simulink model "Full_wave_rectifier_RLload"  (R2015b)
settings: Solver=ode45  StartTime=0.0  StopTime=0.5  FixedStep=50e-6  RelTol=1e-3
InitFcn:
  | Vm=339.4;
libraries: powerlib x12
settings Model: Creator=VENKAT  LastModifiedBy=Nikhil
settings DataIOCC: SaveFormat=Array
settings DebuggingCC: SolverPrmCheckMsg=warning
settings HardwareCC: ProdBitPerPointer=32  ProdLargestAtomicFloat=None  ProdIntDivRoundTo=Undefined  ProdEndianess=Unspecified  ProdWordSize=32  ProdHWDeviceType=32-bit Generic
settings GRTTargetCC: GeneratePreprocessorConditionals=Disable all
settings ConfigComp: CovModelRefEnable=Off  CovSFcnEnable=off

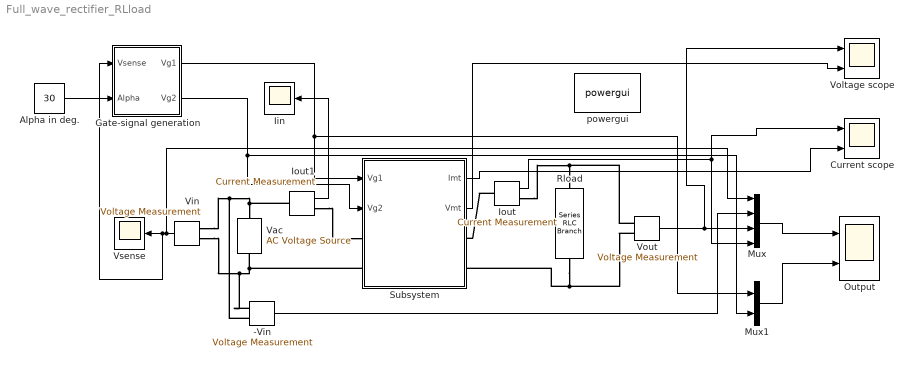
== system Full_wave_rectifier_RLload ==
  -Vin : powerlib/Measurements/Voltage Measurement  PhasorSimulation=off  OutputType=Complex  PSBequivalent=0
  Alpha in deg. : Constant  Value=30
  Current scope : Scope  NumInputPorts=2
  Gate-signal generation : Subsystem
  Iin : Scope
  Iout : powerlib/Measurements/Current Measurement  PhasorSimulation=off  OutputType=Complex  PSBequivalent=0
  Iout1 : powerlib/Measurements/Current Measurement  PhasorSimulation=off  OutputType=Complex  PSBequivalent=0
  Mux : Mux
  Mux1 : Mux  Inputs=2
  Output : Scope  NumInputPorts=2
  Rload : powerlib/Elements/Series RLC Branch  LConnTagsString=__new0  RConnTagsString=__new0  BranchType=RL  Resistance=1  Inductance=1e-2  SetiL0=off  InitialCurrent=0  Capacitance=1e-6  Setx0=off  InitialVoltage=0  Measurements=None
  Subsystem : Subsystem
  Vac : powerlib/Electrical Sources/AC Voltage Source  Amplitude=Vm  Phase=0  Frequency=50  SampleTime=0  Measurements=None  BusType=swing  Pref=10e3  Qref=0  Qmin=-inf  Qmax=+inf
  Vin : powerlib/Measurements/Voltage Measurement  PhasorSimulation=off  OutputType=Complex  PSBequivalent=0
  Voltage scope : Scope  NumInputPorts=2
  Vout : powerlib/Measurements/Voltage Measurement  PhasorSimulation=off  OutputType=Complex  PSBequivalent=0
  Vsense : Scope
  powergui : powerlib/powergui  Priority=1  SimulationMode=Continuous  SolverType=Tustin  SampleTime=50e-6  frequency=60  SPID=on  DisableSnubberDevices=off  DisableRonSwitches=off  DisableVfSwitches=off  SwTol=0  DisplayEquations=off  Interpol=off  ExternalGateDelay=off  methode=off  Ts=0  FunctionMessages=off  echomessages=off  HookPort=off  EnableUseOfTLC=off  x0status=blocks  frequencyindice=50  Pbase=100e6  ErrMax=1e-4  Iterations=50  UnitsV=kV  UnitsW=MW  buscounter=0  RestoreLinks=warning  ResistiveCurrentMeasurement=off  Frange=[0:2:500]  Ylog=off  Xlog=on  ShowGrid=off  save=off  variable=ZData  structure=0  ZoomFFT=off  StartTime=0.0  cycles=1  DisplayStyle=1  fundamental=60  FreqAxis=off  MaxFrequency=1000  frequencyindicesteady=1  RmsSteady=1  display=off
  wires:
  Vin/1 -> Mux/1, Gate-signal generation/1(Vsense), Vsense/1
  Alpha in deg./1 -> Gate-signal generation/2(Alpha)
  Mux/1 -> Output/1
  Gate-signal generation/1(Vg1) -> Mux1/1, Subsystem/1(Vg1)
  Gate-signal generation/2(Vg2) -> Mux1/2, Subsystem/2(Vg2)
  Iout/1 -> Mux/4, Current scope/1
  Vout/1 -> Voltage scope/1, Mux/3
  -Vin/1 -> Mux/2
  Mux1/1 -> Output/2
  Subsystem/1(Imt) -> Current scope/2
  Subsystem/2(Vmt) -> Voltage scope/2
  Iout1/1 -> Iin/1
  connections:
  Vin/LConn1 -- -Vin/LConn2 -- Iout1/LConn1 -- Vac/RConn1
  Rload/RConn1 -- Vout/LConn2 -- Subsystem/RConn2
  Vout/LConn1 -- Iout/RConn1 -- Rload/LConn1
  Vin/LConn2 -- -Vin/LConn1 -- Subsystem/LConn2 -- Vac/LConn1
  Iout/LConn1 -- Subsystem/RConn1
  Iout1/RConn1 -- Subsystem/LConn1

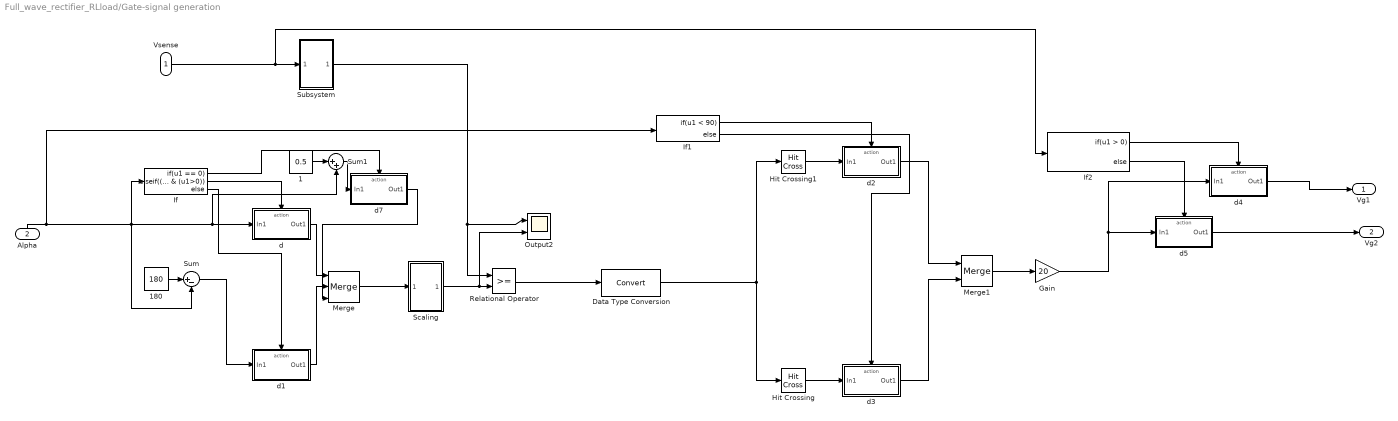
== system Full_wave_rectifier_RLload/Gate-signal generation ==
  Vsense : Inport
  Alpha : Inport  Port=2
  1 : Constant  Value=0.5
  180 : Constant  Value=180
  Data Type Conversion : DataTypeConversion
  Gain : Gain  Gain=20
  Hit Crossing : HitCross  HitCrossingOffset=1e-5  HitCrossingDirection=falling
  Hit Crossing1 : HitCross  HitCrossingDirection=rising
  If : If  IfExpression=u1 == 0  ElseIfExpressions=(u1 < 90) & (u1>0)
  If1 : If  IfExpression=u1 < 90
  If2 : If
  Merge : Merge  Inputs=3
  Merge1 : Merge
  Output2 : Scope  NumInputPorts=2
  Relational Operator : RelationalOperator  OutDataTypeStr=boolean
  Scaling : Subsystem
  Subsystem : Subsystem
  Sum : Sum  Inputs=|+-
  Sum1 : Sum  Inputs=|++
  d : Subsystem  TreatAsAtomicUnit=on
  d1 : Subsystem  TreatAsAtomicUnit=on
  d2 : Subsystem  TreatAsAtomicUnit=on
  d3 : Subsystem  TreatAsAtomicUnit=on
  d4 : Subsystem  TreatAsAtomicUnit=on
  d5 : Subsystem  TreatAsAtomicUnit=on
  d7 : Subsystem  TreatAsAtomicUnit=on
  Vg1 : Outport
  Vg2 : Outport  Port=2
  wires:
  Sum/1 -> d1/1(In1)
  180/1 -> Sum/1
  Alpha/1 -> If1/1, If/1, Sum1/2, d/1(In1), Sum/2
  If/3 -> d1/Action
  d/1(Out1) -> Merge/1
  d1/1(Out1) -> Merge/2
  Relational Operator/1 -> Data Type Conversion/1
  If1/1 -> d2/Action
  If1/2 -> d3/Action
  Data Type Conversion/1 -> Hit Crossing/1, Hit Crossing1/1
  Hit Crossing1/1 -> d2/1(In1)
  Hit Crossing/1 -> d3/1(In1)
  d2/1(Out1) -> Merge1/1
  d3/1(Out1) -> Merge1/2
  Merge1/1 -> Gain/1
  Merge/1 -> Scaling/1(In1)
  Scaling/1(Out1) -> Output2/2, Relational Operator/2
  Vsense/1 -> If2/1, Subsystem/1(In1)
  Subsystem/1(Out2) -> Output2/1, Relational Operator/1
  If2/1 -> d4/Action
  Gain/1 -> d5/1(In1), d4/1(In1)
  d4/1(Out1) -> Vg1/1
  d5/1(Out1) -> Vg2/1
  If2/2 -> d5/Action
  If/2 -> d/Action
  If/1 -> d7/Action
  d7/1(Out1) -> Merge/3
  1/1 -> Sum1/1
  Sum1/1 -> d7/1(In1)

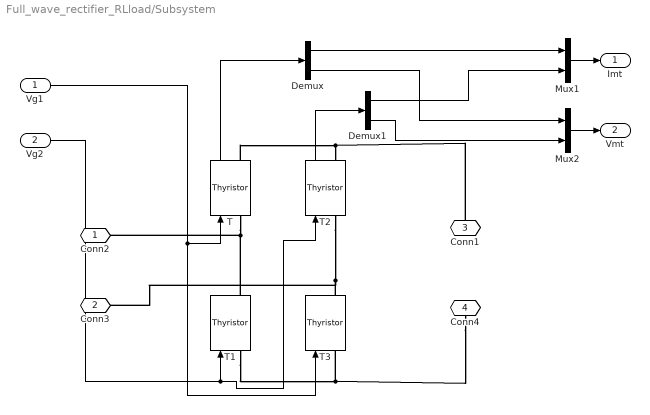
== system Full_wave_rectifier_RLload/Subsystem ==
  Vg1 : Inport
  Vg2 : Inport  Port=2
  Demux : Demux  Outputs=2
  Demux1 : Demux  Outputs=2
  Mux1 : Mux  Inputs=2
  Mux2 : Mux  Inputs=2
  T{,1..3} (4 alike) : powerlib/Power Electronics/Thyristor  Ron=0.001  Lon=0  Vf=0.8  IC=0  Rs=500  Cs=250e-9  Measurements=on
  Conn2 : PMIOPort  Port=1  Side=Left
  Conn3 : PMIOPort  Port=2  Side=Left
  Conn1 : PMIOPort  Port=3  Side=Right
  Conn4 : PMIOPort  Port=4  Side=Right
  Imt : Outport
  Vmt : Outport  Port=2
  wires:
  Vg2/1 -> T1/1, T2/1
  Vg1/1 -> T3/1, T/1
  T/1 -> Demux/1
  T2/1 -> Demux1/1
  Demux/1 -> Mux1/1
  Demux1/1 -> Mux1/2
  Demux/2 -> Mux2/1
  Demux1/2 -> Mux2/2
  Mux1/1 -> Imt/1
  Mux2/1 -> Vmt/1
  connections:
  T1/RConn1 -- Conn2/RConn1 -- T/LConn1
  T1/LConn1 -- Conn4/RConn1 -- T3/LConn1
  T/RConn1 -- Conn1/RConn1 -- T2/RConn1
  T2/LConn1 -- T3/RConn1 -- Conn3/RConn1

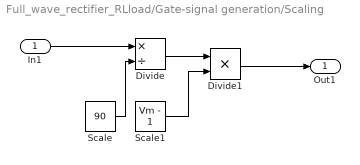
== system Full_wave_rectifier_RLload/Gate-signal generation/Scaling ==
  In1 : Inport
  Divide : Product  Inputs=*/
  Divide1 : Product  Inputs=**
  Scale : Constant  Value=90
  Scale1 : Constant  Value=Vm - 1
  Out1 : Outport
  wires:
  Scale1/1 -> Divide1/2
  Divide1/1 -> Out1/1
  Scale/1 -> Divide/2
  Divide/1 -> Divide1/1
  In1/1 -> Divide/1

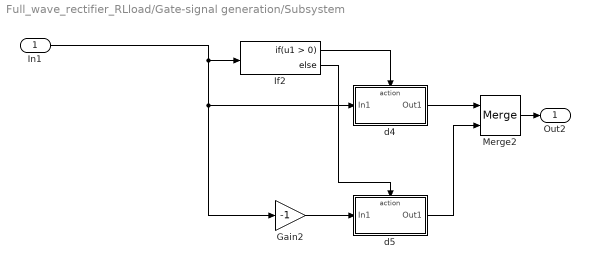
== system Full_wave_rectifier_RLload/Gate-signal generation/Subsystem ==
  In1 : Inport
  Gain2 : Gain  Gain=-1
  If2 : If
  Merge2 : Merge
  d4 : Subsystem  TreatAsAtomicUnit=on
  d5 : Subsystem  TreatAsAtomicUnit=on
  Out2 : Outport
  wires:
  Gain2/1 -> d5/1(In1)
  d5/1(Out1) -> Merge2/2
  d4/1(Out1) -> Merge2/1
  In1/1 -> Gain2/1, d4/1(In1), If2/1
  If2/2 -> d5/Action
  Merge2/1 -> Out2/1
  If2/1 -> d4/Action

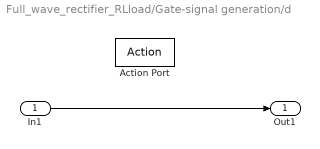
== system Full_wave_rectifier_RLload/Gate-signal generation/d ==
  In1 : Inport
  Action Port : ActionPort  ActionType=elseif
  Out1 : Outport
  wires:
  In1/1 -> Out1/1

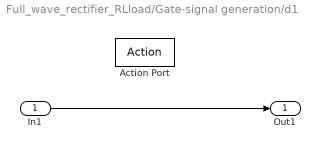
== system Full_wave_rectifier_RLload/Gate-signal generation/d1 ==
  In1 : Inport
  Action Port : ActionPort  ActionType=else
  Out1 : Outport
  wires:
  In1/1 -> Out1/1

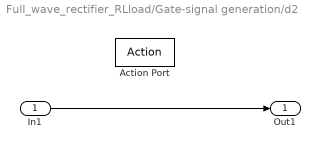
== system Full_wave_rectifier_RLload/Gate-signal generation/d2 ==
  In1 : Inport
  Action Port : ActionPort  ActionType=then
  Out1 : Outport
  wires:
  In1/1 -> Out1/1

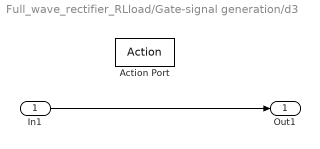
== system Full_wave_rectifier_RLload/Gate-signal generation/d3 ==
  In1 : Inport
  Action Port : ActionPort  ActionType=else
  Out1 : Outport
  wires:
  In1/1 -> Out1/1

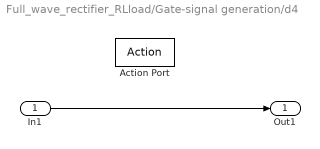
== system Full_wave_rectifier_RLload/Gate-signal generation/d4 ==
  In1 : Inport
  Action Port : ActionPort  ActionType=then
  Out1 : Outport
  wires:
  In1/1 -> Out1/1

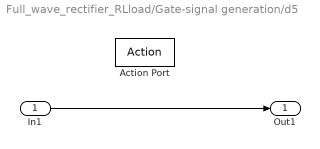
== system Full_wave_rectifier_RLload/Gate-signal generation/d5 ==
  In1 : Inport
  Action Port : ActionPort  ActionType=else
  Out1 : Outport
  wires:
  In1/1 -> Out1/1

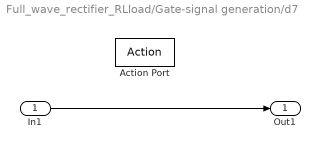
== system Full_wave_rectifier_RLload/Gate-signal generation/d7 ==
  In1 : Inport
  Action Port : ActionPort  ActionType=then
  Out1 : Outport
  wires:
  In1/1 -> Out1/1

== system Full_wave_rectifier_RLload/Gate-signal generation/Subsystem/d4 ==
  In1 : Inport
  Action Port : ActionPort  ActionType=then
  Out1 : Outport
  wires:
  In1/1 -> Out1/1

== system Full_wave_rectifier_RLload/Gate-signal generation/Subsystem/d5 ==
  In1 : Inport
  Action Port : ActionPort  ActionType=else
  Out1 : Outport
  wires:
  In1/1 -> Out1/1
